simulink model "Double_Pendulum_Model"  (R2020b)
settings: Solver=ode4  StartTime=0.0  StopTime=5  FixedStep=0.01  RelTol=1e-3
InitFcn:
  | m11=0.25;
  | m12=0;
  | m21=0.25;
  | m22=0.25;
  | c11=0;
  | c12=0;
  | c21=0;
  | c22=0;
  | k11=9.8;
  | k12=-4.9;
  | k21=0;
  | k22=4.9;
settings Model: Creator=Amir  LastModifiedBy=vahed
settings DataIOCC: ReturnWorkspaceOutputs=off
settings DebuggingCC: ArithmeticOperatorsInVariantConditions=warning
settings SFSimCC: CustomCodeUndefinedFunction=UseInterfaceOnly

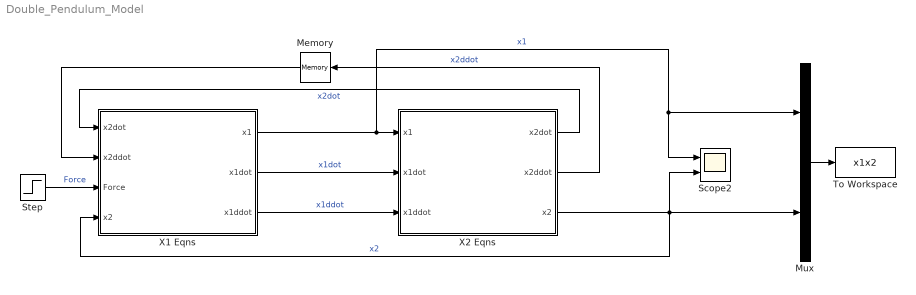
== system Double_Pendulum_Model ==
  Memory : Memory
  Mux : Mux  Inputs=2
  Scope2 : Scope  NumInputPorts=2
  Step : Step  After=0  SampleTime=0
  To Workspace : ToWorkspace  VariableName=x1x2  SaveFormat=Timeseries  SampleTime=-1
  X1 Eqns : Subsystem
  X2 Eqns : Subsystem
  wires:
  Mux/1 -> To Workspace/1
  X1 Eqns/1(x1) -> Scope2/1, Mux/1, X2 Eqns/1(x1)  "x1"
  Step/1 -> X1 Eqns/3(Force)  "Force"
  X2 Eqns/3(x2) -> X1 Eqns/4(x2), Mux/2, Scope2/2  "x2"
  X1 Eqns/2(x1dot) -> X2 Eqns/2(x1dot)  "x1dot"
  X1 Eqns/3(x1ddot) -> X2 Eqns/3(x1ddot)  "x1ddot"
  X2 Eqns/1(x2dot) -> X1 Eqns/1(x2dot)  "x2dot"
  X2 Eqns/2(x2ddot) -> Memory/1  "x2ddot"
  Memory/1 -> X1 Eqns/2(x2ddot)

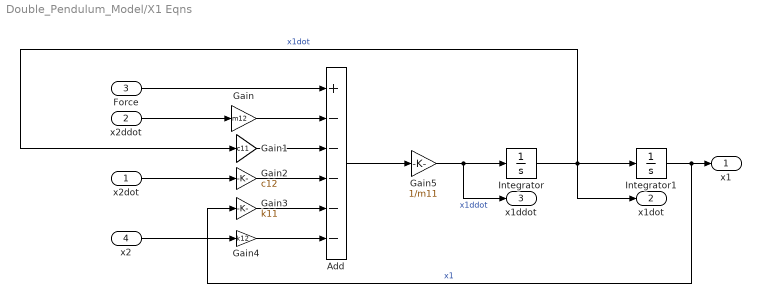
== system Double_Pendulum_Model/X1 Eqns ==
  x2dot : Inport
  x2ddot : Inport  Port=2
  Force : Inport  Port=3
  x2 : Inport  Port=4
  Add : Sum  Inputs=+-----
  Gain : Gain  Gain=m12
  Gain1 : Gain  Gain=c11
  Gain2 : Gain  Gain=c12
  Gain3 : Gain  Gain=k11
  Gain4 : Gain  Gain=k12
  Gain5 : Gain  Gain=1/m11
  Integrator : Integrator
  Integrator1 : Integrator
  x1 : Outport
  x1dot : Outport  Port=2
  x1ddot : Outport  Port=3
  wires:
  Gain1/1 -> Add/3
  Gain2/1 -> Add/4
  Gain5/1 -> x1ddot/1, Integrator/1  "x1ddot"
  Integrator/1 -> x1dot/1, Gain1/1, Integrator1/1  "x1dot"
  Gain/1 -> Add/2
  Add/1 -> Gain5/1
  Gain4/1 -> Add/6
  Gain3/1 -> Add/5
  Force/1 -> Add/1
  x2ddot/1 -> Gain/1
  x2/1 -> Gain4/1
  Integrator1/1 -> Gain3/1, x1/1  "x1"
  x2dot/1 -> Gain2/1

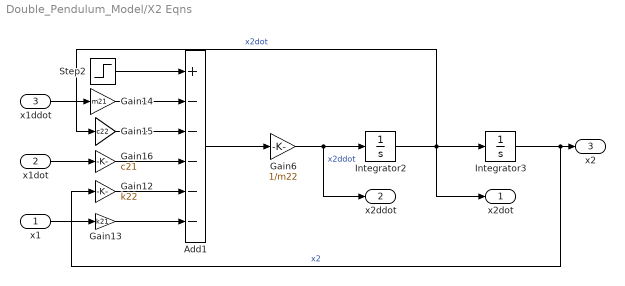
== system Double_Pendulum_Model/X2 Eqns ==
  x1 : Inport
  x1dot : Inport  Port=2
  x1ddot : Inport  Port=3
  Add1 : Sum  Inputs=+-----
  Gain12 : Gain  Gain=k22
  Gain13 : Gain  Gain=k21
  Gain14 : Gain  Gain=m21
  Gain15 : Gain  Gain=c22
  Gain16 : Gain  Gain=c21
  Gain6 : Gain  Gain=1/m22
  Integrator2 : Integrator
  Integrator3 : Integrator  InitialCondition=3*pi/180
  Step2 : Step  After=0  SampleTime=0
  x2dot : Outport
  x2ddot : Outport  Port=2
  x2 : Outport  Port=3
  wires:
  Step2/1 -> Add1/1
  Gain14/1 -> Add1/2
  Integrator2/1 -> Gain15/1, x2dot/1, Integrator3/1  "x2dot"
  Add1/1 -> Gain6/1
  Gain13/1 -> Add1/6
  x1/1 -> Gain13/1
  Gain16/1 -> Add1/4
  Gain12/1 -> Add1/5
  Gain15/1 -> Add1/3
  Gain6/1 -> x2ddot/1, Integrator2/1  "x2ddot"
  Integrator3/1 -> Gain12/1, x2/1  "x2"
  x1dot/1 -> Gain16/1
  x1ddot/1 -> Gain14/1
